simulink model "FaceDet_x4"  (Simulink 7.7)
settings: Solver=FixedStepDiscrete  StartTime=0  StopTime=10  RelTol=1e-3
libraries: simulink x257
(part 5 of 5)

== system FaceDet_x4/FaceDetection/FU/CalcIntegralImg/HorzRunningSum/Accumulator15/UDlyER ==
  note: UnitDelayEnabledResettable
  u : Inport
  E : Inport  Port=2
  R : Inport  Port=3
  FixPt Unit Delay1 : UnitDelay  X0=vinit  SampleTime=tsamp
  ICond : Constant  Value=vinit  OutDataTypeStr=Inherit: Inherit via back propagation
  SwitchEn : MultiPortSwitch  DataPortOrder=Zero-based contiguous  Inputs=2  zeroidx=on
  SwitchRst : MultiPortSwitch  DataPortOrder=Zero-based contiguous  Inputs=2  zeroidx=on
  y : Outport
  wires:
  R/1 -> SwitchRst/1  "Reset"
  SwitchEn/1 -> SwitchRst/2
  u/1 -> SwitchEn/3  "Data"
  E/1 -> SwitchEn/1  "Enable"
  FixPt Unit Delay1/1 -> y/1, SwitchEn/2  "Xold"
  SwitchRst/1 -> FixPt Unit Delay1/1  "Xnew"
  ICond/1 -> SwitchRst/3  "IVal"

== system FaceDet_x4/FaceDetection/FU/CalcIntegralImg/HorzRunningSum/Accumulator16/UDlyER ==
  note: UnitDelayEnabledResettable
  u : Inport
  E : Inport  Port=2
  R : Inport  Port=3
  FixPt Unit Delay1 : UnitDelay  X0=vinit  SampleTime=tsamp
  ICond : Constant  Value=vinit  OutDataTypeStr=Inherit: Inherit via back propagation
  SwitchEn : MultiPortSwitch  DataPortOrder=Zero-based contiguous  Inputs=2  zeroidx=on
  SwitchRst : MultiPortSwitch  DataPortOrder=Zero-based contiguous  Inputs=2  zeroidx=on
  y : Outport
  wires:
  ICond/1 -> SwitchRst/3  "IVal"
  SwitchRst/1 -> FixPt Unit Delay1/1  "Xnew"
  FixPt Unit Delay1/1 -> SwitchEn/2, y/1  "Xold"
  E/1 -> SwitchEn/1  "Enable"
  u/1 -> SwitchEn/3  "Data"
  SwitchEn/1 -> SwitchRst/2
  R/1 -> SwitchRst/1  "Reset"

== system FaceDet_x4/FaceDetection/FU/CalcIntegralImg/HorzRunningSum/Accumulator17/UDlyER ==
  note: UnitDelayEnabledResettable
  u : Inport
  E : Inport  Port=2
  R : Inport  Port=3
  FixPt Unit Delay1 : UnitDelay  X0=vinit  SampleTime=tsamp
  ICond : Constant  Value=vinit  OutDataTypeStr=Inherit: Inherit via back propagation
  SwitchEn : MultiPortSwitch  DataPortOrder=Zero-based contiguous  Inputs=2  zeroidx=on
  SwitchRst : MultiPortSwitch  DataPortOrder=Zero-based contiguous  Inputs=2  zeroidx=on
  y : Outport
  wires:
  R/1 -> SwitchRst/1  "Reset"
  SwitchEn/1 -> SwitchRst/2
  u/1 -> SwitchEn/3  "Data"
  E/1 -> SwitchEn/1  "Enable"
  FixPt Unit Delay1/1 -> y/1, SwitchEn/2  "Xold"
  SwitchRst/1 -> FixPt Unit Delay1/1  "Xnew"
  ICond/1 -> SwitchRst/3  "IVal"

== system FaceDet_x4/FaceDetection/FU/CalcIntegralImg/HorzRunningSum/Accumulator18/UDlyER ==
  note: UnitDelayEnabledResettable
  u : Inport
  E : Inport  Port=2
  R : Inport  Port=3
  FixPt Unit Delay1 : UnitDelay  X0=vinit  SampleTime=tsamp
  ICond : Constant  Value=vinit  OutDataTypeStr=Inherit: Inherit via back propagation
  SwitchEn : MultiPortSwitch  DataPortOrder=Zero-based contiguous  Inputs=2  zeroidx=on
  SwitchRst : MultiPortSwitch  DataPortOrder=Zero-based contiguous  Inputs=2  zeroidx=on
  y : Outport
  wires:
  ICond/1 -> SwitchRst/3  "IVal"
  SwitchRst/1 -> FixPt Unit Delay1/1  "Xnew"
  FixPt Unit Delay1/1 -> SwitchEn/2, y/1  "Xold"
  E/1 -> SwitchEn/1  "Enable"
  u/1 -> SwitchEn/3  "Data"
  SwitchEn/1 -> SwitchRst/2
  R/1 -> SwitchRst/1  "Reset"

== system FaceDet_x4/FaceDetection/FU/CalcIntegralImg/HorzRunningSum/Accumulator19/UDlyER ==
  note: UnitDelayEnabledResettable
  u : Inport
  E : Inport  Port=2
  R : Inport  Port=3
  FixPt Unit Delay1 : UnitDelay  X0=vinit  SampleTime=tsamp
  ICond : Constant  Value=vinit  OutDataTypeStr=Inherit: Inherit via back propagation
  SwitchEn : MultiPortSwitch  DataPortOrder=Zero-based contiguous  Inputs=2  zeroidx=on
  SwitchRst : MultiPortSwitch  DataPortOrder=Zero-based contiguous  Inputs=2  zeroidx=on
  y : Outport
  wires:
  R/1 -> SwitchRst/1  "Reset"
  SwitchEn/1 -> SwitchRst/2
  u/1 -> SwitchEn/3  "Data"
  E/1 -> SwitchEn/1  "Enable"
  FixPt Unit Delay1/1 -> y/1, SwitchEn/2  "Xold"
  SwitchRst/1 -> FixPt Unit Delay1/1  "Xnew"
  ICond/1 -> SwitchRst/3  "IVal"

== system FaceDet_x4/FaceDetection/FU/CalcIntegralImg/HorzRunningSum/Accumulator2/UDlyER ==
  note: UnitDelayEnabledResettable
  u : Inport
  E : Inport  Port=2
  R : Inport  Port=3
  FixPt Unit Delay1 : UnitDelay  X0=vinit  SampleTime=tsamp
  ICond : Constant  Value=vinit  OutDataTypeStr=Inherit: Inherit via back propagation
  SwitchEn : MultiPortSwitch  DataPortOrder=Zero-based contiguous  Inputs=2  zeroidx=on
  SwitchRst : MultiPortSwitch  DataPortOrder=Zero-based contiguous  Inputs=2  zeroidx=on
  y : Outport
  wires:
  ICond/1 -> SwitchRst/3  "IVal"
  SwitchRst/1 -> FixPt Unit Delay1/1  "Xnew"
  FixPt Unit Delay1/1 -> SwitchEn/2, y/1  "Xold"
  E/1 -> SwitchEn/1  "Enable"
  u/1 -> SwitchEn/3  "Data"
  SwitchEn/1 -> SwitchRst/2
  R/1 -> SwitchRst/1  "Reset"

== system FaceDet_x4/FaceDetection/FU/CalcIntegralImg/HorzRunningSum/Accumulator20/UDlyER ==
  note: UnitDelayEnabledResettable
  u : Inport
  E : Inport  Port=2
  R : Inport  Port=3
  FixPt Unit Delay1 : UnitDelay  X0=vinit  SampleTime=tsamp
  ICond : Constant  Value=vinit  OutDataTypeStr=Inherit: Inherit via back propagation
  SwitchEn : MultiPortSwitch  DataPortOrder=Zero-based contiguous  Inputs=2  zeroidx=on
  SwitchRst : MultiPortSwitch  DataPortOrder=Zero-based contiguous  Inputs=2  zeroidx=on
  y : Outport
  wires:
  ICond/1 -> SwitchRst/3  "IVal"
  SwitchRst/1 -> FixPt Unit Delay1/1  "Xnew"
  FixPt Unit Delay1/1 -> SwitchEn/2, y/1  "Xold"
  E/1 -> SwitchEn/1  "Enable"
  u/1 -> SwitchEn/3  "Data"
  SwitchEn/1 -> SwitchRst/2
  R/1 -> SwitchRst/1  "Reset"

== system FaceDet_x4/FaceDetection/FU/CalcIntegralImg/HorzRunningSum/Accumulator21/UDlyER ==
  note: UnitDelayEnabledResettable
  u : Inport
  E : Inport  Port=2
  R : Inport  Port=3
  FixPt Unit Delay1 : UnitDelay  X0=vinit  SampleTime=tsamp
  ICond : Constant  Value=vinit  OutDataTypeStr=Inherit: Inherit via back propagation
  SwitchEn : MultiPortSwitch  DataPortOrder=Zero-based contiguous  Inputs=2  zeroidx=on
  SwitchRst : MultiPortSwitch  DataPortOrder=Zero-based contiguous  Inputs=2  zeroidx=on
  y : Outport
  wires:
  R/1 -> SwitchRst/1  "Reset"
  SwitchEn/1 -> SwitchRst/2
  u/1 -> SwitchEn/3  "Data"
  E/1 -> SwitchEn/1  "Enable"
  FixPt Unit Delay1/1 -> y/1, SwitchEn/2  "Xold"
  SwitchRst/1 -> FixPt Unit Delay1/1  "Xnew"
  ICond/1 -> SwitchRst/3  "IVal"

== system FaceDet_x4/FaceDetection/FU/CalcIntegralImg/HorzRunningSum/Accumulator22/UDlyER ==
  note: UnitDelayEnabledResettable
  u : Inport
  E : Inport  Port=2
  R : Inport  Port=3
  FixPt Unit Delay1 : UnitDelay  X0=vinit  SampleTime=tsamp
  ICond : Constant  Value=vinit  OutDataTypeStr=Inherit: Inherit via back propagation
  SwitchEn : MultiPortSwitch  DataPortOrder=Zero-based contiguous  Inputs=2  zeroidx=on
  SwitchRst : MultiPortSwitch  DataPortOrder=Zero-based contiguous  Inputs=2  zeroidx=on
  y : Outport
  wires:
  ICond/1 -> SwitchRst/3  "IVal"
  SwitchRst/1 -> FixPt Unit Delay1/1  "Xnew"
  FixPt Unit Delay1/1 -> SwitchEn/2, y/1  "Xold"
  E/1 -> SwitchEn/1  "Enable"
  u/1 -> SwitchEn/3  "Data"
  SwitchEn/1 -> SwitchRst/2
  R/1 -> SwitchRst/1  "Reset"

== system FaceDet_x4/FaceDetection/FU/CalcIntegralImg/HorzRunningSum/Accumulator23/UDlyER ==
  note: UnitDelayEnabledResettable
  u : Inport
  E : Inport  Port=2
  R : Inport  Port=3
  FixPt Unit Delay1 : UnitDelay  X0=vinit  SampleTime=tsamp
  ICond : Constant  Value=vinit  OutDataTypeStr=Inherit: Inherit via back propagation
  SwitchEn : MultiPortSwitch  DataPortOrder=Zero-based contiguous  Inputs=2  zeroidx=on
  SwitchRst : MultiPortSwitch  DataPortOrder=Zero-based contiguous  Inputs=2  zeroidx=on
  y : Outport
  wires:
  R/1 -> SwitchRst/1  "Reset"
  SwitchEn/1 -> SwitchRst/2
  u/1 -> SwitchEn/3  "Data"
  E/1 -> SwitchEn/1  "Enable"
  FixPt Unit Delay1/1 -> y/1, SwitchEn/2  "Xold"
  SwitchRst/1 -> FixPt Unit Delay1/1  "Xnew"
  ICond/1 -> SwitchRst/3  "IVal"

== system FaceDet_x4/FaceDetection/FU/CalcIntegralImg/HorzRunningSum/Accumulator3/UDlyER ==
  note: UnitDelayEnabledResettable
  u : Inport
  E : Inport  Port=2
  R : Inport  Port=3
  FixPt Unit Delay1 : UnitDelay  X0=vinit  SampleTime=tsamp
  ICond : Constant  Value=vinit  OutDataTypeStr=Inherit: Inherit via back propagation
  SwitchEn : MultiPortSwitch  DataPortOrder=Zero-based contiguous  Inputs=2  zeroidx=on
  SwitchRst : MultiPortSwitch  DataPortOrder=Zero-based contiguous  Inputs=2  zeroidx=on
  y : Outport
  wires:
  R/1 -> SwitchRst/1  "Reset"
  SwitchEn/1 -> SwitchRst/2
  u/1 -> SwitchEn/3  "Data"
  E/1 -> SwitchEn/1  "Enable"
  FixPt Unit Delay1/1 -> y/1, SwitchEn/2  "Xold"
  SwitchRst/1 -> FixPt Unit Delay1/1  "Xnew"
  ICond/1 -> SwitchRst/3  "IVal"

== system FaceDet_x4/FaceDetection/FU/CalcIntegralImg/HorzRunningSum/Accumulator4/UDlyER ==
  note: UnitDelayEnabledResettable
  u : Inport
  E : Inport  Port=2
  R : Inport  Port=3
  FixPt Unit Delay1 : UnitDelay  X0=vinit  SampleTime=tsamp
  ICond : Constant  Value=vinit  OutDataTypeStr=Inherit: Inherit via back propagation
  SwitchEn : MultiPortSwitch  DataPortOrder=Zero-based contiguous  Inputs=2  zeroidx=on
  SwitchRst : MultiPortSwitch  DataPortOrder=Zero-based contiguous  Inputs=2  zeroidx=on
  y : Outport
  wires:
  ICond/1 -> SwitchRst/3  "IVal"
  SwitchRst/1 -> FixPt Unit Delay1/1  "Xnew"
  FixPt Unit Delay1/1 -> SwitchEn/2, y/1  "Xold"
  E/1 -> SwitchEn/1  "Enable"
  u/1 -> SwitchEn/3  "Data"
  SwitchEn/1 -> SwitchRst/2
  R/1 -> SwitchRst/1  "Reset"

== system FaceDet_x4/FaceDetection/FU/CalcIntegralImg/HorzRunningSum/Accumulator5/UDlyER ==
  note: UnitDelayEnabledResettable
  u : Inport
  E : Inport  Port=2
  R : Inport  Port=3
  FixPt Unit Delay1 : UnitDelay  X0=vinit  SampleTime=tsamp
  ICond : Constant  Value=vinit  OutDataTypeStr=Inherit: Inherit via back propagation
  SwitchEn : MultiPortSwitch  DataPortOrder=Zero-based contiguous  Inputs=2  zeroidx=on
  SwitchRst : MultiPortSwitch  DataPortOrder=Zero-based contiguous  Inputs=2  zeroidx=on
  y : Outport
  wires:
  R/1 -> SwitchRst/1  "Reset"
  SwitchEn/1 -> SwitchRst/2
  u/1 -> SwitchEn/3  "Data"
  E/1 -> SwitchEn/1  "Enable"
  FixPt Unit Delay1/1 -> y/1, SwitchEn/2  "Xold"
  SwitchRst/1 -> FixPt Unit Delay1/1  "Xnew"
  ICond/1 -> SwitchRst/3  "IVal"

== system FaceDet_x4/FaceDetection/FU/CalcIntegralImg/HorzRunningSum/Accumulator6/UDlyER ==
  note: UnitDelayEnabledResettable
  u : Inport
  E : Inport  Port=2
  R : Inport  Port=3
  FixPt Unit Delay1 : UnitDelay  X0=vinit  SampleTime=tsamp
  ICond : Constant  Value=vinit  OutDataTypeStr=Inherit: Inherit via back propagation
  SwitchEn : MultiPortSwitch  DataPortOrder=Zero-based contiguous  Inputs=2  zeroidx=on
  SwitchRst : MultiPortSwitch  DataPortOrder=Zero-based contiguous  Inputs=2  zeroidx=on
  y : Outport
  wires:
  ICond/1 -> SwitchRst/3  "IVal"
  SwitchRst/1 -> FixPt Unit Delay1/1  "Xnew"
  FixPt Unit Delay1/1 -> SwitchEn/2, y/1  "Xold"
  E/1 -> SwitchEn/1  "Enable"
  u/1 -> SwitchEn/3  "Data"
  SwitchEn/1 -> SwitchRst/2
  R/1 -> SwitchRst/1  "Reset"

== system FaceDet_x4/FaceDetection/FU/CalcIntegralImg/HorzRunningSum/Accumulator7/UDlyER ==
  note: UnitDelayEnabledResettable
  u : Inport
  E : Inport  Port=2
  R : Inport  Port=3
  FixPt Unit Delay1 : UnitDelay  X0=vinit  SampleTime=tsamp
  ICond : Constant  Value=vinit  OutDataTypeStr=Inherit: Inherit via back propagation
  SwitchEn : MultiPortSwitch  DataPortOrder=Zero-based contiguous  Inputs=2  zeroidx=on
  SwitchRst : MultiPortSwitch  DataPortOrder=Zero-based contiguous  Inputs=2  zeroidx=on
  y : Outport
  wires:
  R/1 -> SwitchRst/1  "Reset"
  SwitchEn/1 -> SwitchRst/2
  u/1 -> SwitchEn/3  "Data"
  E/1 -> SwitchEn/1  "Enable"
  FixPt Unit Delay1/1 -> y/1, SwitchEn/2  "Xold"
  SwitchRst/1 -> FixPt Unit Delay1/1  "Xnew"
  ICond/1 -> SwitchRst/3  "IVal"

== system FaceDet_x4/FaceDetection/FU/CalcIntegralImg/HorzRunningSum/Accumulator8/UDlyER ==
  note: UnitDelayEnabledResettable
  u : Inport
  E : Inport  Port=2
  R : Inport  Port=3
  FixPt Unit Delay1 : UnitDelay  X0=vinit  SampleTime=tsamp
  ICond : Constant  Value=vinit  OutDataTypeStr=Inherit: Inherit via back propagation
  SwitchEn : MultiPortSwitch  DataPortOrder=Zero-based contiguous  Inputs=2  zeroidx=on
  SwitchRst : MultiPortSwitch  DataPortOrder=Zero-based contiguous  Inputs=2  zeroidx=on
  y : Outport
  wires:
  ICond/1 -> SwitchRst/3  "IVal"
  SwitchRst/1 -> FixPt Unit Delay1/1  "Xnew"
  FixPt Unit Delay1/1 -> SwitchEn/2, y/1  "Xold"
  E/1 -> SwitchEn/1  "Enable"
  u/1 -> SwitchEn/3  "Data"
  SwitchEn/1 -> SwitchRst/2
  R/1 -> SwitchRst/1  "Reset"

== system FaceDet_x4/FaceDetection/FU/CalcIntegralImg/HorzRunningSum/Accumulator9/UDlyER ==
  note: UnitDelayEnabledResettable
  u : Inport
  E : Inport  Port=2
  R : Inport  Port=3
  FixPt Unit Delay1 : UnitDelay  X0=vinit  SampleTime=tsamp
  ICond : Constant  Value=vinit  OutDataTypeStr=Inherit: Inherit via back propagation
  SwitchEn : MultiPortSwitch  DataPortOrder=Zero-based contiguous  Inputs=2  zeroidx=on
  SwitchRst : MultiPortSwitch  DataPortOrder=Zero-based contiguous  Inputs=2  zeroidx=on
  y : Outport
  wires:
  R/1 -> SwitchRst/1  "Reset"
  SwitchEn/1 -> SwitchRst/2
  u/1 -> SwitchEn/3  "Data"
  E/1 -> SwitchEn/1  "Enable"
  FixPt Unit Delay1/1 -> y/1, SwitchEn/2  "Xold"
  SwitchRst/1 -> FixPt Unit Delay1/1  "Xnew"
  ICond/1 -> SwitchRst/3  "IVal"

== matlab function FaceDetection/FU/FaceDetectionControl ==
  data: En output double; Rst output double; LatchIdxLatch output double; LatchIdxExt output double; NodeWeightsCtrlRdAdr output double; NodeWeightsCtrlWrAdr output double; NodeWeightsCtrlEn output double; NodeWeightsExt output uint(12) size=1; FeatureDataLatch output double; FeatureDataExt output double; WeakTreshLatch output double; WeakTreshExt output double; StrongTreshLatch output double; StrongTreshExt output double
function [En, Rst, LatchIdxLatch, LatchIdxExt, NodeWeightsCtrlRdAdr, NodeWeightsCtrlWrAdr, ...
          NodeWeightsCtrlEn, NodeWeightsExt, FeatureDataLatch, FeatureDataExt, ...
          WeakTreshLatch, WeakTreshExt, StrongTreshLatch, StrongTreshExt] ...
          = FaceDetCtrl( )

persistent En_r Rst_r LatchIdxLatch_r LatchIdxExt_r NodeWeightsCtrlRdAdr_r NodeWeightsCtrlWrAdr_r;
persistent NodeWeightsCtrlEn_r NodeWeightsExt_r FeatureDataLatch_r FeatureDataExt_r;
persistent WeakTreshLatch_r WeakTreshExt_r StrongTreshLatch_r StrongTreshExt_r;
        
if( isempty( En_r ) ),
    En_r = false;
end

if( isempty( Rst_r ) ),
    Rst_r = false;
end

if( isempty( LatchIdxLatch_r ) ),
    LatchIdxLatch_r = false;
end

if( isempty( LatchIdxExt_r ) ),
    LatchIdxExt_r = fi( 0, 0, 20, 0, 'overflowmode', 'wrap' );
end

if( isempty( NodeWeightsCtrlRdAdr_r ) ),
    NodeWeightsCtrlRdAdr_r = fi( 0, 0, 5, 0, 'overflowmode', 'wrap' );
end

if( isempty( NodeWeightsCtrlWrAdr_r ) ),
    NodeWeightsCtrlWrAdr_r = fi( 0, 0, 5, 0, 'overflowmode', 'wrap' );
end

if( isempty( NodeWeightsCtrlEn_r ) ),
    NodeWeightsCtrlEn_r = false;
end

if( isempty( NodeWeightsExt_r ) ),
    NodeWeightsExt_r = fi( 0, 0, 12, 0, 'overflowmode', 'wrap' );
end

if( isempty( FeatureDataLatch_r ) ),
    FeatureDataLatch_r = false;
end

if( isempty( FeatureDataExt_r ) ),
    FeatureDataExt_r = fi( 0, 0, 17, 0, 'overflowmode', 'wrap' );
end

if( isempty( WeakTreshLatch_r ) ),
    WeakTreshLatch_r = false;
end

if( isempty( WeakTreshExt_r ) ),
    WeakTreshExt_r = fi( 0, 0, 25, 0, 'overflowmode', 'wrap' );
end

if( isempty( StrongTreshLatch_r ) ),
    StrongTreshLatch_r = false;
end

if( isempty( StrongTreshExt_r ) ),
    StrongTreshExt_r = fi( 0, 0, 21, 0, 'overflowmode', 'wrap' );
end

En = En_r;
Rst = Rst_r;
LatchIdxLatch = LatchIdxLatch_r;
LatchIdxExt = LatchIdxExt_r;
NodeWeightsCtrlRdAdr = NodeWeightsCtrlRdAdr_r;
NodeWeightsCtrlWrAdr = NodeWeightsCtrlWrAdr_r;
NodeWeightsCtrlEn = NodeWeightsCtrlEn_r;
NodeWeightsExt = NodeWeightsExt_r;
FeatureDataLatch = FeatureDataLatch_r;
FeatureDataExt = FeatureDataExt_r;
WeakTreshLatch = WeakTreshLatch_r;
WeakTreshExt = WeakTreshExt_r;
StrongTreshLatch = StrongTreshLatch_r;
StrongTreshExt = StrongTreshExt_r;

En_r = xor( En_r, true );
Rst_r = xor( Rst_r, true );
LatchIdxLatch_r = xor( LatchIdxLatch_r, true );
LatchIdxExt_r = fi( LatchIdxExt_r + fi( 1, 0, 20, 0, 'overflowmode', 'wrap' ), 0, 20, 0, 'overflowmode', 'wrap' );
NodeWeightsCtrlRdAdr_r = fi( NodeWeightsCtrlRdAdr_r + fi( 1, 0, 5, 0, 'overflowmode', 'wrap' ), 0, 5, 0, 'overflowmode', 'wrap' );
NodeWeightsCtrlWrAdr_r = fi( NodeWeightsCtrlWrAdr_r + fi( 1, 0, 5, 0, 'overflowmode', 'wrap' ), 0, 5, 0, 'overflowmode', 'wrap' );
NodeWeightsCtrlEn_r = xor( NodeWeightsCtrlEn_r, true );
NodeWeightsExt_r = fi( NodeWeightsExt_r + fi( 1, 0, 12, 0, 'overflowmode', 'wrap' ), 0, 12, 0, 'overflowmode', 'wrap' );
FeatureDataLatch_r = xor( FeatureDataLatch_r, true );
FeatureDataExt_r = fi( FeatureDataExt_r + fi( 1, 0, 17, 0, 'overflowmode', 'wrap' ), 0, 17, 0, 'overflowmode', 'wrap' );
WeakTreshLatch_r = xor( WeakTreshLatch_r, true );
WeakTreshExt_r = fi( WeakTreshExt_r + fi( 1, 0, 25, 0, 'overflowmode', 'wrap' ), 0, 25, 0, 'overflowmode', 'wrap' );
StrongTreshLatch_r = xor( StrongTreshLatch_r, true );
StrongTreshExt_r = fi( StrongTreshExt_r + fi( 1, 0, 21, 0, 'overflowmode', 'wrap' ), 0, 21, 0, 'overflowmode', 'wrap' );
